simulink model "P_sim"  (R2022b)
settings: Solver=VariableStepAuto  StartTime=0.0  StopTime=100  RelTol=1e-3
values from neighbouring files (symbols this model uses):
  k1a = k1(i)    [P.m]
settings Model: Creator=zuzanna  LastModifiedBy=zuzanna

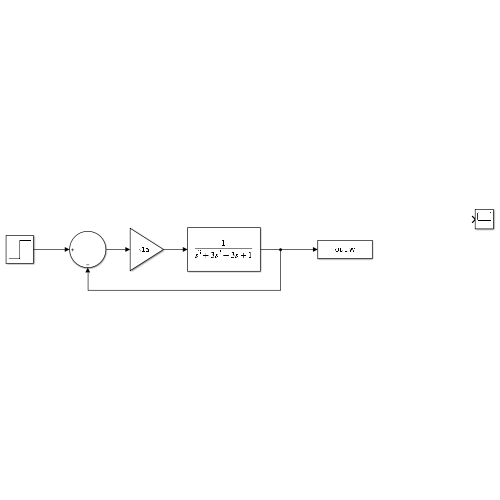
[thumbnail: Simulink's stored preview of the top-level diagram]
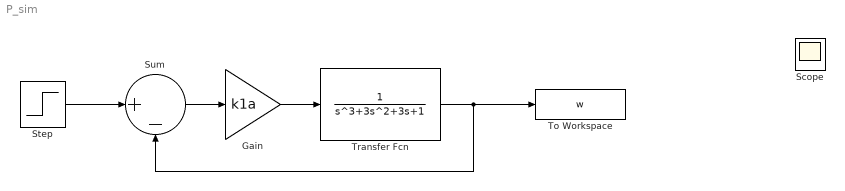
== system P_sim ==
  Gain : Gain  Gain=k1a
  Scope : Scope
  Step : Step  SampleTime=0
  Sum : Sum  Inputs=|+-
  To Workspace : ToWorkspace  VariableName=w  SampleTime=-1
  Transfer Fcn : TransferFcn  Denominator=[1 3 3 1]
  wires:
  Sum/1 -> Gain/1
  Transfer Fcn/1 -> Sum/2, To Workspace/1
  Gain/1 -> Transfer Fcn/1
  Step/1 -> Sum/1
